simulink model "Euler_eqs"  (R2018b)
settings: Solver=ode45  StartTime=0.0  StopTime=100  RelTol=1e-8  EnableMultiTasking=on
settings Model: Creator=jsb12221  LastModifiedBy=aloisia
settings DataIOCC: LimitDataPoints=on  SaveFormat=Array  SignalLoggingSaveFormat=ModelDataLogs
settings OptimizationCC: ExpressionDepthLimit=2147483647  LifeSpan=inf
settings DebuggingCC: UnderspecifiedInitializationDetection=Classic  MergeDetectMultiDrivingBlocksExec=none  FcnCallInpInsideContextMsg=warning  UnknownTsInhSupMsg=none  StateNameClashWarn=warning  LibraryContextMissingDiagnostic=none  SFUnexpectedBacktrackingDiag=warning  SFNoUnconditionalDefaultTransitionDiag=warning  SFExecutionAtInitializationDiag=none
settings HardwareCC: ProdBitPerPointer=32  ProdBitPerSizeT=32  ProdBitPerPtrDiffT=32  ProdLargestAtomicFloat=None  ProdIntDivRoundTo=Undefined  ProdEndianess=Unspecified  ProdWordSize=32  ProdHWDeviceType=32-bit Generic
settings ModelReferenceCC: PropagateSignalLabelsOutOfModel=off
settings SFSimCC: SimUseLocalCustomCode=off
settings RTWCC: RTWUseLocalCustomCode=off
settings CodeAppCC: StateflowObjectComments=on
settings GRTTargetCC: TargetLangStandard=C89/C90 (ANSI)  GeneratePreprocessorConditionals=Disable all
settings ConfigComp: CovMetricSettings=dw  CovHtmlReporting=on  CovSaveCumulativeToWorkspaceVar=on  CovSaveSingleToWorkspaceVar=on  CovExternalEMLEnable=off

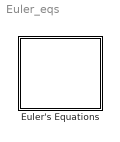
== system Euler_eqs ==
  "Euler's Equations " : Subsystem

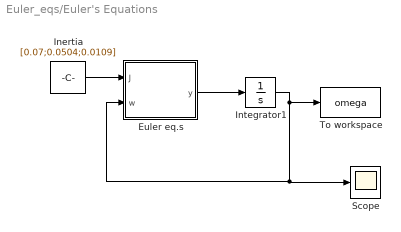
== system Euler_eqs/Euler's Equations  ==
  Euler eq.s : MATLAB Function  TreatAsAtomicUnit=on
  Inertia : Constant  Value=[0.07;0.0504;0.0109]
  Integrator1 : Integrator  InitialCondition=[0.45; 0.52; 0.55]
  "Scope " : Scope
  To workspace : ToWorkspace  VariableName=omega  SampleTime=-1
  wires:
  Integrator1/1 -> To workspace/1, Euler eq.s/2(w), "Scope "/1
  Inertia/1 -> Euler eq.s/1(J)
  Euler eq.s/1(y) -> Integrator1/1

== matlab function Euler_eqs/Euler's Equations /Euler eq.s ==
  data: J input; w input; y output
function y = euler_eqs(J,w)

J1=J(1);
J2=J(2);
J3=J(3);

w_dot = zeros(3,1);

c1 = ((J2-J3)/J1);
c2 = ((J3-J1)/J2);
c3 = ((J1-J2)/J3);

w_dot(1) = c1*w(2)*w(3);
w_dot(2) = c2*w(1)*w(3) ;
w_dot(3) = c3*w(2)*w(1);

y=w_dot;
